simulink model "BackWheelCarLike"  (Simulink 9.2)
settings: Solver=ode5  StartTime=0.0  StopTime=5  FixedStep=Ts  RelTol=1e-3  EnableMultiTasking=on
values from neighbouring files (symbols this model uses):
  a = 49*cm_unit    (= 0.49)    [parameters.m]
  b = 0.300    (= 0.3)    [Fusion 2.m]    (also in parameters.m = 0.27)
  phi_init = deg2rad(0)    [Initial_posture.m]
  psi_init = deg2rad(0)    [Initial_posture.m]
  rw = 0.060    (= 0.06)    [Fusion 2.m]    (also in parameters.m = 0.065)
  Ts = 5*1e-2    (= 0.05)    [parameters.m]
  v_init = 1    [Initial_posture.m]
  xCr_init = 0    [Initial_posture.m]
  yCr_init = 0    [Initial_posture.m]
undefined symbols (not defined in the file or in its folder): DiscIntNeverNeededParam
libraries: simulink x2
settings Model: Creator=nasralla  LastModifiedBy=Mahesh
settings DataIOCC: LimitDataPoints=off
settings OptimizationCC: ExpressionDepthLimit=2147483647  InitFltsAndDblsToZero=on
settings DebuggingCC: SaveWithParameterizedLinksMsg=none  SolverPrmCheckMsg=warning
settings GRTTargetCC: TargetFcnLib=ansi_tfl_tmw.mat  GeneratePreprocessorConditionals=Use local settings

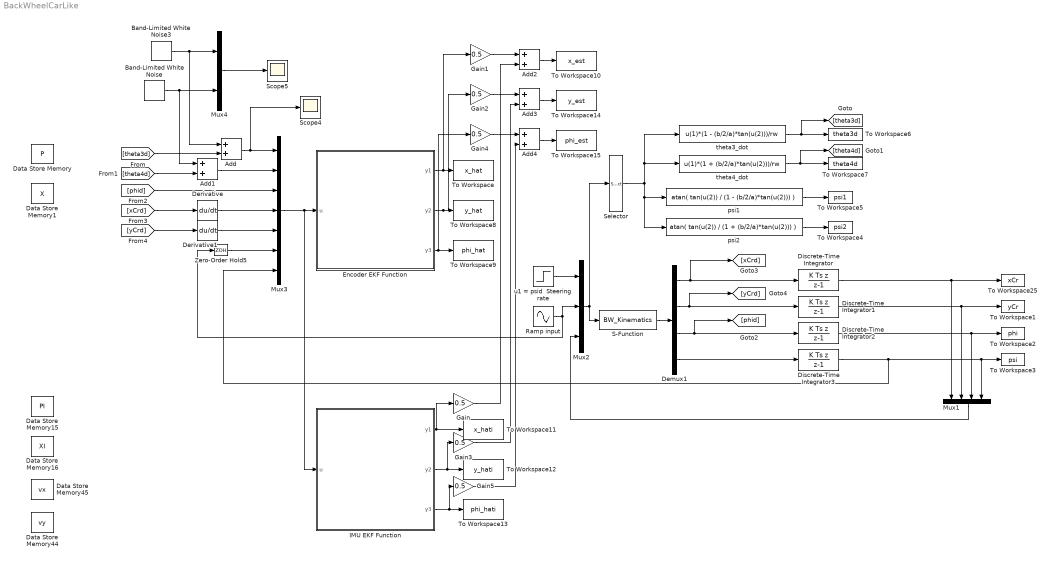
== system BackWheelCarLike ==
  Add{,1..4} (5 alike) : Sum
  Band-Limited White Noise : simulink/Sources/Band-Limited White Noise  Cov=[0.01]  Ts=Ts  seed=[12334]
  Band-Limited White Noise3 : simulink/Sources/Band-Limited White Noise  Cov=[0.01]  Ts=Ts  seed=[12334]
  Data Store Memory : DataStoreMemory  DataStoreName=P  ReadBeforeWriteMsg=warning  WriteAfterWriteMsg=warning  WriteAfterReadMsg=warning  InitialValue=P  ShowAdditionalParam=off  OutDataTypeStr=double
  Data Store Memory1 : DataStoreMemory  DataStoreName=X  ReadBeforeWriteMsg=warning  WriteAfterWriteMsg=warning  WriteAfterReadMsg=warning  InitialValue=X  ShowAdditionalParam=off  OutDataTypeStr=double
  Data Store Memory15 : DataStoreMemory  DataStoreName=PI  ReadBeforeWriteMsg=warning  WriteAfterWriteMsg=warning  WriteAfterReadMsg=warning  InitialValue=PI  ShowAdditionalParam=off  OutDataTypeStr=double
  Data Store Memory16 : DataStoreMemory  DataStoreName=XI  ReadBeforeWriteMsg=warning  WriteAfterWriteMsg=warning  WriteAfterReadMsg=warning  InitialValue=XI  ShowAdditionalParam=off  OutDataTypeStr=double
  Data Store Memory44 : DataStoreMemory  DataStoreName=vy  ReadBeforeWriteMsg=warning  WriteAfterWriteMsg=warning  WriteAfterReadMsg=warning  InitialValue=vy  ShowAdditionalParam=off  OutDataTypeStr=double
  Data Store Memory45 : DataStoreMemory  DataStoreName=vx  ReadBeforeWriteMsg=warning  WriteAfterWriteMsg=warning  WriteAfterReadMsg=warning  InitialValue=vx  ShowAdditionalParam=off  OutDataTypeStr=double
  Demux1 : Demux
  Derivative : Derivative
  Derivative1 : Derivative
  Discrete-Time Integrator : DiscreteIntegrator  IntegratorMethod=Integration: Backward Euler  InitialCondition=xCr_init  SampleTime=-1  ICPrevOutput=DiscIntNeverNeededParam  ICPrevScaledInput=DiscIntNeverNeededParam
  Discrete-Time Integrator1 : DiscreteIntegrator  IntegratorMethod=Integration: Backward Euler  InitialCondition=yCr_init  SampleTime=-1  ICPrevOutput=DiscIntNeverNeededParam  ICPrevScaledInput=DiscIntNeverNeededParam
  Discrete-Time Integrator2 : DiscreteIntegrator  IntegratorMethod=Integration: Backward Euler  InitialCondition=phi_init  SampleTime=-1  ICPrevOutput=DiscIntNeverNeededParam  ICPrevScaledInput=DiscIntNeverNeededParam
  Discrete-Time Integrator3 : DiscreteIntegrator  IntegratorMethod=Integration: Backward Euler  InitialCondition=psi_init  SampleTime=-1  ICPrevOutput=DiscIntNeverNeededParam  ICPrevScaledInput=DiscIntNeverNeededParam
  Encoder EKF Function : MATLAB Function  TreatAsAtomicUnit=on
  Gain{,1..5} (6 alike) : Gain  Gain=0.5
  IMU EKF Function : MATLAB Function  TreatAsAtomicUnit=on
  Mux1 : Mux
  Mux2 : Mux  Inputs=3
  Mux3 : Mux  Inputs=7
  Mux4 : Mux  Inputs=2
  Ramp input : Sin  Amplitude=0  Bias=v_init  Frequency=.2*pi  SampleTime=0
  S-Function : S-Function  FunctionName=BW_Kinematics  SFunctionDeploymentMode=off  EnableBusSupport=off
  Scope4 : Scope
  Scope5 : Scope
  Selector : Selector  InputPortWidth=6  IndexOptions=Index vector (dialog)  Indices=[2 6]  OutputSizes=1
  To Workspace : ToWorkspace  VariableName=x_hat  SampleTime=-1
      settings: Save2DSignal=2-D array (concatenate along first dimension)
  To Workspace1 : ToWorkspace  VariableName=yCr  SampleTime=-1
  To Workspace10 : ToWorkspace  VariableName=x_est  SampleTime=-1
      settings: Save2DSignal=2-D array (concatenate along first dimension)
  To Workspace11 : ToWorkspace  VariableName=x_hati  SampleTime=-1
      settings: Save2DSignal=2-D array (concatenate along first dimension)
  To Workspace12 : ToWorkspace  VariableName=y_hati  SampleTime=-1
      settings: Save2DSignal=2-D array (concatenate along first dimension)
  To Workspace13 : ToWorkspace  VariableName=phi_hati  SampleTime=-1
      settings: Save2DSignal=2-D array (concatenate along first dimension)
  To Workspace14 : ToWorkspace  VariableName=y_est  SampleTime=-1
      settings: Save2DSignal=2-D array (concatenate along first dimension)
  To Workspace15 : ToWorkspace  VariableName=phi_est  SampleTime=-1
      settings: Save2DSignal=2-D array (concatenate along first dimension)
  To Workspace2 : ToWorkspace  VariableName=phi  SampleTime=-1
  To Workspace25 : ToWorkspace  VariableName=xCr  SampleTime=-1
  To Workspace3 : ToWorkspace  VariableName=psi  SampleTime=-1
  To Workspace4 : ToWorkspace  VariableName=psi2  SampleTime=-1
  To Workspace5 : ToWorkspace  VariableName=psi1  SampleTime=-1
  To Workspace6 : ToWorkspace  VariableName=theta3d  SampleTime=-1
  To Workspace7 : ToWorkspace  VariableName=theta4d  SampleTime=-1
  To Workspace8 : ToWorkspace  VariableName=y_hat  SampleTime=-1
      settings: Save2DSignal=2-D array (concatenate along first dimension)
  To Workspace9 : ToWorkspace  VariableName=phi_hat  SampleTime=-1
      settings: Save2DSignal=2-D array (concatenate along first dimension)
  Zero-Order Hold5 : ZeroOrderHold  SampleTime=-1
  psi1 : Fcn  Expr=atan( tan(u(2)) / (1 - (b/2/a)*tan(u(2))) )
  psi2 : Fcn  Expr=atan( tan(u(2)) / (1 + (b/2/a)*tan(u(2))) )
  theta3_dot : Fcn  Expr=u(1)*(1 - (b/2/a)*tan(u(2)))/rw
  theta4_dot : Fcn  Expr=u(1)*(1 + (b/2/a)*tan(u(2)))/rw
  u1 = psid  Steering rate : Step  After=0.0873  SampleTime=0
  wires:
  S-Function/1 -> Demux1/1
  Mux2/1 -> S-Function/1, Selector/1
  Mux1/1 -> Mux2/3
  Selector/1 -> psi2/1, psi1/1, theta4_dot/1, theta3_dot/1
  psi2/1 -> To Workspace4/1
  psi1/1 -> To Workspace5/1
  theta4_dot/1 -> [theta4d], To Workspace7/1
  theta3_dot/1 -> [theta3d], To Workspace6/1
  Encoder EKF Function/2(y2) -> Gain2/1, To Workspace8/1
  Encoder EKF Function/3(y3) -> To Workspace9/1, Gain4/1
  Encoder EKF Function/1(y1) -> Gain1/1, To Workspace/1
  [theta3d] -> Add/2
  [theta4d] -> Add1/2
  Mux4/1 -> Scope5/1
  IMU EKF Function/1(y1) -> Gain/1, To Workspace11/1
  IMU EKF Function/2(y2) -> Gain3/1, To Workspace12/1
  IMU EKF Function/3(y3) -> Gain5/1, To Workspace13/1
  Mux3/1 -> IMU EKF Function/1(u), Encoder EKF Function/1(u)
  [xCrd] -> Derivative/1
  u1 = psid  Steering rate/1 -> Mux2/1
  Zero-Order Hold5/1 -> Mux3/6
  Discrete-Time Integrator3/1 -> Mux3/7, To Workspace3/1, Mux1/4
  Ramp input/1 -> Mux2/2, Zero-Order Hold5/1
  Discrete-Time Integrator/1 -> Mux1/1, To Workspace25/1
  Demux1/1 -> Discrete-Time Integrator/1, [xCrd]
  Discrete-Time Integrator1/1 -> Mux1/2, To Workspace1/1
  Demux1/2 -> [yCrd], Discrete-Time Integrator1/1
  Band-Limited White Noise3/1 -> Add/1, Mux4/1
  Band-Limited White Noise/1 -> Add1/1, Mux4/2
  Discrete-Time Integrator2/1 -> Mux1/3, To Workspace2/1
  Demux1/3 -> [phid], Discrete-Time Integrator2/1
  Demux1/4 -> Discrete-Time Integrator3/1
  [yCrd] -> Derivative1/1
  Add1/1 -> Mux3/2
  Add/1 -> Scope4/1, Mux3/1
  [phid] -> Mux3/3
  Derivative/1 -> Mux3/4
  Derivative1/1 -> Mux3/5
  Gain/1 -> Add2/2
  Gain1/1 -> Add2/1
  Add2/1 -> To Workspace10/1
  Gain2/1 -> Add3/1
  Add3/1 -> To Workspace14/1
  Gain3/1 -> Add3/2
  Add4/1 -> To Workspace15/1
  Gain4/1 -> Add4/1
  Gain5/1 -> Add4/2

== matlab function IMU EKF Function ==
  settings: updateMethod=DISCRETE
  data: u input double; y1 output double; y2 output double; y3 output double; PI data_store_memory double; XI data_store_memory double; vx data_store_memory double; vy data_store_memory double
function [y1,y2,y3]= DataFusion(u)

dt=0.05;          %time interval
%rw=0.065;         %wheel rad
%b=0.2700;    %wheel distance measured with error at t
a=0.49;

Q=eye(3)
R=diag([1 1 1]);  %measurement covariance matrix

global PI
global XI
global vx
global vy

Bah = 0;        % x acceleration measurement Bias, TBD by calibration
Bal = 0;        % y acceleration measurement Bias, TBD by calibration
Bg = 0;        % Angular velocity measurement Bias, TBD by calibration

vi=u(6);
psii=u(7);

Ah=  u(4);    % measured with scale error from IMU at t
Al=  u(5);    % measured with scale error from IMU at t
W=  u(3);   % measured with scale error from IMU at t
ah=Ah-Bah;
al=Al-Bal;
% Rotation from (h,l) to (x,y) is to be applied here
% phig=XI(3);
% acc=[cos(phig) -sin(phig); sin(phig) cos(phig)]*[ah; al]; %don't comment out in actual program
% ax=acc(1) %don't comment out in actual program
% ay=acc(2)  %don't comment out in actual program

ax=ah; % comment out in actual program
ay=al; % comment out in actual program


vx = vx + ax*dt;
vy = vy + ay*dt;

%% Sensor model
phi=XI(3);
Xi=XI;
w=W-Bg;
Xi = eye(3)*Xi + [vx*dt ; vy*dt ; w*dt ];
Yi = eye(3)*Xi;


%% Kalman filter starts
XI = eye(3)*XI + [vi*cos(phi)*dt; vi*sin(phi)*dt; (vi*tan(psii)*dt)/a];

A = [1 0 -vi*sin(phi)*dt; 0 1 vi*cos(phi)*dt; 0 0 1];

PI = A*PI*A'+Q;

C = eye(3);

K = PI*C'/(C*PI*C'+R);

XI = XI + K*(Yi-C*XI);

PI = (eye(3)-K*C)*PI;

%% Outputs

y1 = XI(1);
y2 = XI(2);
y3 = XI(3);

%% for next time-step

== matlab function Encoder EKF Function ==
  settings: updateMethod=DISCRETE
  data: u input double; y1 output double; y2 output double; y3 output double; X data_store_memory double; P data_store_memory double
function [y1,y2,y3]= DataFusion(u)


dt=0.05;          %time interval
rw=0.065;         %wheel rad
b=0.2700;    %wheel distance measured with error at t
a=0.49;

Q=eye(3)
R=diag([1 1 1]);  %measurement covariance matrix

global P
global X
%global vl
%global vr
%global v    %input
%global psi  %input

v=u(6);
psi=u(7);
dtheta3=u(1);
dtheta4=u(2);
vl=rw*dtheta3;
vr=rw*dtheta4;


%% Sensor Model
phi=X(3);
Xe=X;
Xe = eye(3)*Xe + [0.5*(vr+vl)*dt*cos(phi); 0.5*(vr+vl)*dt*sin(phi);((vr-vl)*dt)/b ];
Ye = eye(3)*Xe;

%% Kalman filter starts

X = eye(3)*X + [v*cos(phi)*dt; v*sin(phi)*dt; (v*tan(psi)*dt)/a];

A = [1 0 -v*sin(phi)*dt; 0 1 v*cos(phi)*dt; 0 0 1];

P = A*P*A'+Q;

C = eye(3);

K = P*C'/(C*P*C'+R);

X = X + K*(Ye-C*X);

P = (eye(3)-K*C)*P;

%% Outputs

y1 = X(1);
y2 = X(2);
y3 = X(3);

%% for next time-step
